simulink model "ControlRocketAngleGyroWind"  (R2022b)
settings: Solver=ode45  StartTime=0.0  StopTime=100  RelTol=1e-5
PostLoadFcn:
  | flightControlCallback('initializeParameters', bdroot, '3DOF', 0);
InitFcn:
  | flightControlCallback('runSim', bdroot);
undefined symbols (not defined in the file or in its folder): DiscIntNeverNeededParam, F, Light, MIL
libraries: aerolibasang x6, simulink_extras x4, shared3dof x1, aerolibanim x1, simulink x1, aerolibtransform2 x1, aerolibutil x1, slpidlib x1, aerolibwind2 x1
(part 2 of 2)

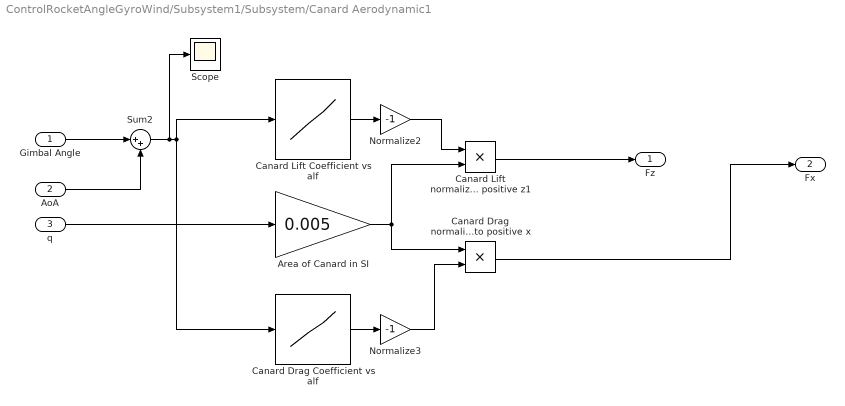
== system ControlRocketAngleGyroWind/Subsystem1/Subsystem/Canard Aerodynamic1 ==
  Gimbal Angle : Inport
  AoA : Inport  Port=2
  q : Inport  Port=3
  Area of Canard in SI : Gain  Gain=0.005
  Canard Drag Coefficient vs alf : Lookup_n-D  NumberOfTableDimensions=1  BreakpointsForDimension1=|  Table=|  InternalRulePriority=Speed  RndMeth=Simplest
      BreakpointsForDimension1=|
      | [-6
      | -5.9
      | -5.8
      | -5.7
      | -5.6
      | -5.5
      | -5.4
      | -5.3
      | -5.2
      | -5.1
      | -5
      | -4.9
      | -4.8
      | -4.7
      | -4.6
      | -4.5
      | -4.4
      | -4.3
      | -4.2
      | -4.1
      | -4
      | -3.9
      | -3.8
      | -3.7
      | -3.6
      | -3.5
      | -3.4
      | -3.3
      | -3.2
      | -3.1
      | -3
      | -2.9
      | -2.8
      | -2.7
      | -2.6
      | -2.4
      | -2.3
      | -2.2
      | -2.1
      | -2
      | -1.9
      | -1.8
      | -1.7
      | -1.6
      | -1.5
      | -1.4
      | -1.3
      | -1.2
      | -1.1
      | -1
      | -0.9
      | -0.8
      | -0.7
      | -0.6
      | -0.5
      | -0.4
      | -0.3
      | -0.2
      | -0.1
      | 0
      | 0.1
      | 0.2
      | 0.3
      | 0.4
      | 0.5
      | 0.6
      | 0.7
      | 0.8
      | 0.9
      | 1
      | 1.1
      | 1.2
      | 1.3
      | 1.4
      | 1.5
      | 1.6
      | 1.7
      | 1.8
      | 1.9
      | 2
      | 2.1
      | 2.2
      | 2.3
      | 2.4
      | 2.5
      | 2.6
      | 2.7
      | 2.8
      | 2.9
      | 3
      | 3.1
      | 3.2
      | 3.3
      | 3.4
      | 3.5
      | 3.6
      | 3.7
      | 3.8
      | 3.9
      | 4
      | 4.1
      | 4.2
      | 4.3
      | 4.4
      | 4.5
      | 4.6
      | 4.7
      | 4.8
      | 4.9
      | 5
      | 5.1
      | 5.2
      | 5.3
      | 5.4
      | 5.5
      | 5.6
      | 5.7
      | 5.8
      | 5.9
      | 6]
      Table=|
      | [0.04364
      | 0.04148
      | 0.03935
      | 0.03724
      | 0.03517
      | 0.03314
      | 0.03118
      | 0.02935
      | 0.02764
      | 0.02597
      | 0.02431
      | 0.02272
      | 0.02125
      | 0.01988
      | 0.01863
      | 0.01752
      | 0.01655
      | 0.01573
      | 0.01489
      | 0.01373
      | 0.01297
      | 0.01255
      | 0.01218
      | 0.01173
      | 0.0113
      | 0.01092
      | 0.01063
      | 0.01009
      | 0.0098
      | 0.0096
      | 0.00942
      | 0.00909
      | 0.00891
      | 0.00868
      | 0.00844
      | 0.00786
      | 0.00753
      | 0.00719
      | 0.00689
      | 0.00663
      | 0.00637
      | 0.00613
      | 0.00593
      | 0.00573
      | 0.00555
      | 0.00538
      | 0.00522
      | 0.00508
      | 0.00495
      | 0.00484
      | 0.00475
      | 0.00469
      | 0.00465
      | 0.00462
      | 0.00462
      | 0.00463
      | 0.00464
      | 0.00465
      | 0.00465
      | 0.00465
      | 0.00465
      | 0.00465
      | 0.00464
      | 0.00463
      | 0.00462
      | 0.00462
      | 0.00465
      | 0.00469
      | 0.00475
      | 0.00484
      | 0.00495
      | 0.00508
      | 0.00522
      | 0.00538
      | 0.00555
      | 0.00573
      | 0.00593
      | 0.00613
      | 0.00637
      | 0.00663
      | 0.00689
      | 0.00719
      | 0.00752
      | 0.00786
      | 0.00817
      | 0.00844
      | 0.00868
      | 0.00891
      | 0.00908
      | 0.00942
      | 0.00961
      | 0.0098
      | 0.01008
      | 0.01063
      | 0.01092
      | 0.0113
      | 0.01173
      | 0.01217
      | 0.01254
      | 0.01297
      | 0.01373
      | 0.0149
      | 0.01572
      | 0.01655
      | 0.01752
      | 0.01863
      | 0.01988
      | 0.02125
      | 0.02273
      | 0.02432
      | 0.02598
      | 0.02764
      | 0.02935
      | 0.03119
      | 0.03316
      | 0.03518
      | 0.03725
      | 0.03936
      | 0.0415
      | 0.04366
      | ]
  Canard Drag normalized to positive x : Product
  Canard Lift Coefficient vs alf : Lookup_n-D  NumberOfTableDimensions=1  BreakpointsForDimension1=|  Table=|  InternalRulePriority=Speed  RndMeth=Simplest
      BreakpointsForDimension1=|
      | [-6
      | -5.9
      | -5.8
      | -5.7
      | -5.6
      | -5.5
      | -5.4
      | -5.3
      | -5.2
      | -5.1
      | -5
      | -4.9
      | -4.8
      | -4.7
      | -4.6
      | -4.5
      | -4.4
      | -4.3
      | -4.2
      | -4.1
      | -4
      | -3.9
      | -3.8
      | -3.7
      | -3.6
      | -3.5
      | -3.4
      | -3.3
      | -3.2
      | -3.1
      | -3
      | -2.9
      | -2.8
      | -2.7
      | -2.6
      | -2.4
      | -2.3
      | -2.2
      | -2.1
      | -2
      | -1.9
      | -1.8
      | -1.7
      | -1.6
      | -1.5
      | -1.4
      | -1.3
      | -1.2
      | -1.1
      | -1
      | -0.9
      | -0.8
      | -0.7
      | -0.6
      | -0.5
      | -0.4
      | -0.3
      | -0.2
      | -0.1
      | 0
      | 0.1
      | 0.2
      | 0.3
      | 0.4
      | 0.5
      | 0.6
      | 0.7
      | 0.8
      | 0.9
      | 1
      | 1.1
      | 1.2
      | 1.3
      | 1.4
      | 1.5
      | 1.6
      | 1.7
      | 1.8
      | 1.9
      | 2
      | 2.1
      | 2.2
      | 2.3
      | 2.4
      | 2.5
      | 2.6
      | 2.7
      | 2.8
      | 2.9
      | 3
      | 3.1
      | 3.2
      | 3.3
      | 3.4
      | 3.5
      | 3.6
      | 3.7
      | 3.8
      | 3.9
      | 4
      | 4.1
      | 4.2
      | 4.3
      | 4.4
      | 4.5
      | 4.6
      | 4.7
      | 4.8
      | 4.9
      | 5
      | 5.1
      | 5.2
      | 5.3
      | 5.4
      | 5.5
      | 5.6
      | 5.7
      | 5.8
      | 5.9
      | 6]
      Table=|
      | [-0.6705
      | -0.6674
      | -0.6637
      | -0.6595
      | -0.6547
      | -0.6492
      | -0.6428
      | -0.6357
      | -0.628
      | -0.6204
      | -0.6127
      | -0.6045
      | -0.5957
      | -0.5863
      | -0.5762
      | -0.5657
      | -0.5547
      | -0.5432
      | -0.5319
      | -0.5218
      | -0.5109
      | -0.4992
      | -0.4873
      | -0.4757
      | -0.4642
      | -0.4525
      | -0.4407
      | -0.43
      | -0.4184
      | -0.4064
      | -0.3945
      | -0.383
      | -0.3711
      | -0.3595
      | -0.3479
      | -0.3254
      | -0.3144
      | -0.3035
      | -0.2924
      | -0.2812
      | -0.27
      | -0.2588
      | -0.2475
      | -0.2363
      | -0.2251
      | -0.2139
      | -0.2027
      | -0.1916
      | -0.1806
      | -0.1698
      | -0.1592
      | -0.1488
      | -0.1369
      | -0.1201
      | -0.1027
      | -0.0839
      | -0.0632
      | -0.0417
      | -0.0212
      | 0
      | 0.0212
      | 0.0417
      | 0.0633
      | 0.0839
      | 0.1027
      | 0.1202
      | 0.137
      | 0.1487
      | 0.1591
      | 0.1698
      | 0.1806
      | 0.1916
      | 0.2026
      | 0.2138
      | 0.225
      | 0.2362
      | 0.2475
      | 0.2588
      | 0.27
      | 0.2811
      | 0.2923
      | 0.3034
      | 0.3144
      | 0.3253
      | 0.3365
      | 0.3479
      | 0.3594
      | 0.3711
      | 0.383
      | 0.3944
      | 0.4064
      | 0.4183
      | 0.4299
      | 0.4406
      | 0.4525
      | 0.4641
      | 0.4756
      | 0.4873
      | 0.4992
      | 0.5109
      | 0.5218
      | 0.5319
      | 0.5433
      | 0.5547
      | 0.5657
      | 0.5763
      | 0.5863
      | 0.5958
      | 0.6046
      | 0.6128
      | 0.6204
      | 0.6281
      | 0.6358
      | 0.643
      | 0.6493
      | 0.6548
      | 0.6596
      | 0.6638
      | 0.6675
      | 0.6706]
  Canard Lift normalized to positive z1 : Product
  Normalize2 : Gain  Gain=-1
  Normalize3 : Gain  Gain=-1
  Scope : Scope
  Sum2 : Sum  Inputs=|++
  Fz : Outport
  Fx : Outport  Port=2
  wires:
  Area of Canard in SI/1 -> Canard Drag normalized to positive x/1, Canard Lift normalized to positive z1/2
  Canard Drag Coefficient vs alf/1 -> Normalize3/1
  Canard Drag normalized to positive x/1 -> Fx/1
  Normalize2/1 -> Canard Lift normalized to positive z1/1
  Sum2/1 -> Scope/1, Canard Drag Coefficient vs alf/1, Canard Lift Coefficient vs alf/1
  Normalize3/1 -> Canard Drag normalized to positive x/2
  Canard Lift Coefficient vs alf/1 -> Normalize2/1
  Canard Lift normalized to positive z1/1 -> Fz/1
  Gimbal Angle/1 -> Sum2/1
  q/1 -> Area of Canard in SI/1
  AoA/1 -> Sum2/2
